simulink model "MAGLEV_StateSpace_szabalyozo"  (Simulink 7.4)
settings: Solver=ode45  StartTime=0.0  StopTime=15  FixedStep=0.01  RelTol=1e-3
undefined symbols (not defined in the file): C, F, G, g, H, K, L0, m, magnitude, Nu, Nx, Q, R, u0, x01, x02, x03
settings Model: Creator=Fodi  LastModifiedBy=Fodi

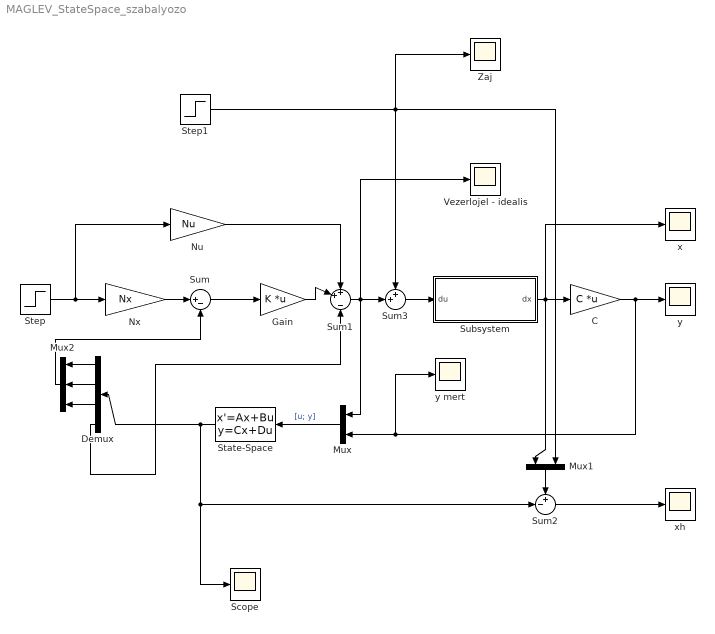
== system MAGLEV_StateSpace_szabalyozo ==
  C : Gain  Gain=C  Multiplication=Matrix(K*u)  ParameterDataType=fixdt(1, 16)  ParameterScaling=2^0  OutDataType=fixdt(1, 16)  OutScaling=2^0
  Demux : Demux
  Gain : Gain  Gain=K  Multiplication=Matrix(K*u)  ParameterDataType=fixdt(1, 16)  ParameterScaling=2^0  OutDataType=fixdt(1, 16)  OutScaling=2^0
  Mux : Mux  Inputs=2
  Mux1 : Mux  Inputs=2
  Mux2 : Mux  Inputs=3
  Nu : Gain  Gain=Nu  ParameterDataType=fixdt(1, 16)  ParameterScaling=2^0  OutDataType=fixdt(1, 16)  OutScaling=2^0
  Nx : Gain  Gain=Nx  ParameterDataType=fixdt(1, 16)  ParameterScaling=2^0  OutDataType=fixdt(1, 16)  OutScaling=2^0
  Scope : Scope
      settings: SaveName=xb
  State-Space : StateSpace  A=F  B=[H G]  C=eye(size(F))  D=zeros(size(F,1),size([H G],2))
  Step : Step  Time=0  After=0.001  SampleTime=0
  Step1 : Step  Time=2  After=0  SampleTime=0
  Subsystem : Subsystem
  Sum : Sum  Inputs=|+-  OutDataType=fixdt(1, 16)  OutScaling=2^0
  Sum1 : Sum  Inputs=++|-  OutDataType=fixdt(1, 16)  OutScaling=2^0
  Sum2 : Sum  Inputs=+-|  OutDataType=fixdt(1, 16)  OutScaling=2^0
  Sum3 : Sum  Inputs=++|  OutDataType=fixdt(1, 16)  OutScaling=2^0
  Vezerlojel - idealis : Scope
      settings: TimeRange=10  YMin=-1  YMax=3  SaveName=u
  Zaj : Scope
      settings: SaveName=ScopeData2
  x : Scope
      settings: SaveName=x
  xh : Scope
      settings: TimeRange=10  YMin=-0.02  YMax=0.12
  y : Scope
      settings: TimeRange=10  YMin=0  YMax=0.0025  SaveName=y
  y mert : Scope
      settings: TimeRange=5  YMin=0  YMax=0.003  SaveName=ym
  wires:
  Step/1 -> Nx/1, Nu/1
  Nx/1 -> Sum/1
  Nu/1 -> Sum1/1
  Gain/1 -> Sum1/2
  Sum/1 -> Gain/1
  Sum1/1 -> Mux/1, Sum3/2, Vezerlojel - idealis/1
  Subsystem/1(dx) -> C/1, Mux1/1, x/1
  State-Space/1 -> Demux/1, Sum2/2, Scope/1
  Mux/1 -> State-Space/1  "[u; y]"
  Step1/1 -> Sum3/1, Mux1/2, Zaj/1
  Sum3/1 -> Subsystem/1(du)
  Mux1/1 -> Sum2/1
  Mux2/1 -> Sum/2
  Demux/4 -> Sum1/3
  Demux/1 -> Mux2/1
  Demux/2 -> Mux2/2
  Demux/3 -> Mux2/3
  Sum2/1 -> xh/1
  C/1 -> y/1, Mux/2, y mert/1

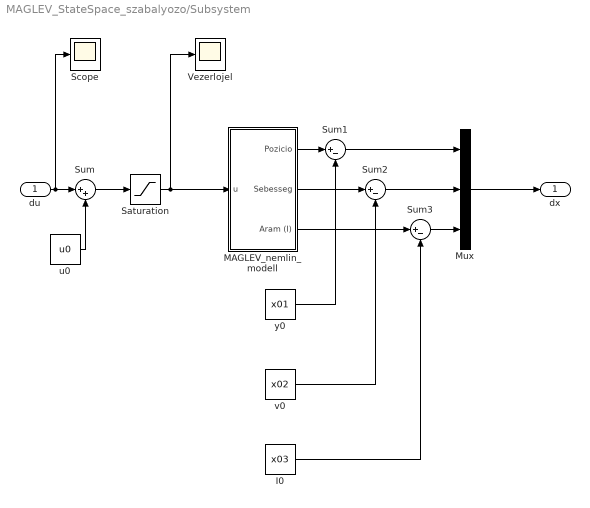
== system MAGLEV_StateSpace_szabalyozo/Subsystem ==
  du : Inport  OutDataType=fixdt(1, 16)  OutScaling=2^0
  I0 : Constant  Value=x03  OutDataType=fixdt(1, 16)  OutScaling=2^0
  MAGLEV_nemlin_modell : Subsystem
  Mux : Mux  Inputs=3
  Saturation : Saturate  UpperLimit=30  LowerLimit=-30  OutDataType=fixdt(1, 16)  OutScaling=2^0
  Scope : Scope
  Sum : Sum  Inputs=|++  OutDataType=fixdt(1, 16)  OutScaling=2^0
  Sum1 : Sum  Inputs=|+-  OutDataType=fixdt(1, 16)  OutScaling=2^0
  Sum2 : Sum  Inputs=|+-  OutDataType=fixdt(1, 16)  OutScaling=2^0
  Sum3 : Sum  Inputs=|+-  OutDataType=fixdt(1, 16)  OutScaling=2^0
  Vezerlojel : Scope
      settings: TimeRange=10  YMin=11  YMax=16  SaveName=ScopeData3
  u0 : Constant  Value=u0  OutDataType=fixdt(1, 16)  OutScaling=2^0
  v0 : Constant  Value=x02  OutDataType=fixdt(1, 16)  OutScaling=2^0
  y0 : Constant  Value=x01  OutDataType=fixdt(1, 16)  OutScaling=2^0
  dx : Outport  OutDataType=fixdt(1, 16)  OutScaling=2^0
  wires:
  y0/1 -> Sum1/2
  v0/1 -> Sum2/2
  I0/1 -> Sum3/2
  MAGLEV_nemlin_modell/3(Aram (I)) -> Sum3/1
  Sum3/1 -> Mux/3
  Sum2/1 -> Mux/2
  Sum1/1 -> Mux/1
  u0/1 -> Sum/2
  Mux/1 -> dx/1
  MAGLEV_nemlin_modell/2(Sebesseg) -> Sum2/1
  MAGLEV_nemlin_modell/1(Pozicio) -> Sum1/1
  du/1 -> Scope/1, Sum/1
  Sum/1 -> Saturation/1
  Saturation/1 -> MAGLEV_nemlin_modell/1(u), Vezerlojel/1

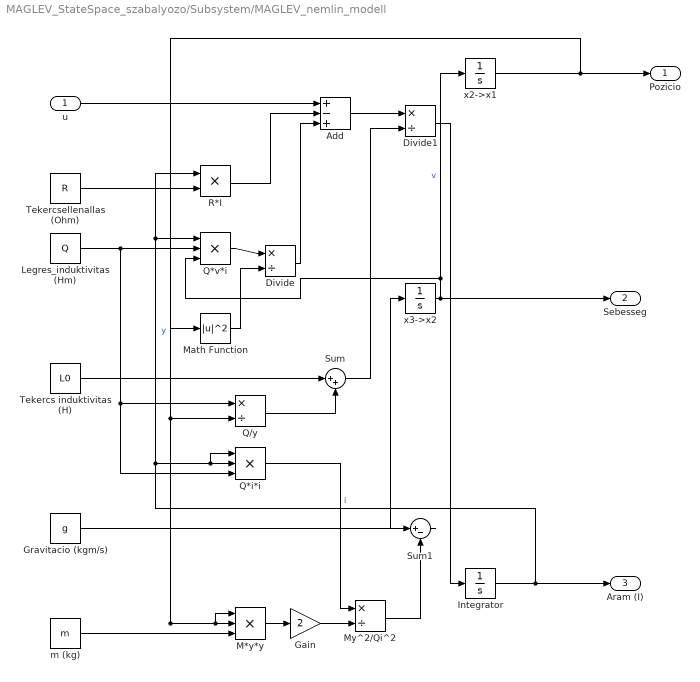
== system MAGLEV_StateSpace_szabalyozo/Subsystem/MAGLEV_nemlin_modell ==
  u : Inport  Tag=v  OutDataType=fixdt(1, 16)  OutScaling=2^0
  Add : Sum  Inputs=+-+  OutDataType=fixdt(1, 16)  OutScaling=2^-10
  Divide : Product  Inputs=*/  OutDataType=fixdt(1, 16)  OutScaling=2^-10
  Divide1 : Product  Inputs=*/  OutDataType=fixdt(1, 16)  OutScaling=2^-10
  Gain : Gain  Gain=2  ParameterDataType=fixdt(1, 16)  ParameterScaling=2^0  OutDataType=fixdt(1, 16)  OutScaling=2^0
  Gravitacio (kgm/s) : Constant  Value=g  OutDataType=fixdt(1, 16)  OutScaling=2^0
  Integrator : Integrator  InitialCondition=x03
  Legres_induktivitas (Hm) : Constant  Value=Q  OutDataType=fixdt(1, 16)  OutScaling=2^0
  M*y*y : Product  Inputs=3  OutDataType=fixdt(1, 16)  OutScaling=2^0  RndMeth=Zero
  Math Function : Math  Operator=magnitude^2  OutDataType=fixdt(1, 16)  OutScaling=2^0  SaturateOnIntegerOverflow=on
  My^2/Qi^2 : Product  Inputs=*/  OutDataType=fixdt(1, 16)  OutScaling=2^-10
  Q*i*i : Product  Inputs=3  OutDataType=fixdt(1, 16)  OutScaling=2^0  RndMeth=Zero
  Q*v*i : Product  Inputs=3  OutDataType=fixdt(1, 16)  OutScaling=2^0  RndMeth=Zero
  Q/y : Product  Inputs=*/  OutDataType=fixdt(1, 16)  OutScaling=2^-10
  R*I : Product  OutDataType=fixdt(1, 16)  OutScaling=2^0  RndMeth=Zero
  Sum : Sum  Inputs=|++  OutDataType=fixdt(1, 16)  OutScaling=2^0
  Sum1 : Sum  Inputs=|+-  OutDataType=fixdt(1, 16)  OutScaling=2^0
  Tekercs induktivitas (H) : Constant  Value=L0  OutDataType=fixdt(1, 16)  OutScaling=2^0
  Tekercsellenallas (Ohm) : Constant  Value=R  OutDataType=fixdt(1, 16)  OutScaling=2^0
  m (kg) : Constant  Value=m  OutDataType=fixdt(1, 16)  OutScaling=2^0
  x2->x1 : Integrator  InitialCondition=x01
  x3->x2 : Integrator  InitialCondition=0.01
  Pozicio : Outport  OutDataType=fixdt(1, 16)  OutScaling=2^0
  Sebesseg : Outport  Port=2  OutDataType=fixdt(1, 16)  OutScaling=2^0
  Aram (I) : Outport  Port=3  OutDataType=fixdt(1, 16)  OutScaling=2^0
  wires:
  x2->x1/1 -> Pozicio/1, Q/y/2, Math Function/1, M*y*y/2, M*y*y/1  "y"
  Sum1/1 -> x3->x2/1
  Gravitacio (kgm/s)/1 -> Sum1/1
  My^2/Qi^2/1 -> Sum1/2
  Gain/1 -> My^2/Qi^2/2
  M*y*y/1 -> Gain/1
  Sum/1 -> Divide1/2
  Tekercs induktivitas (H)/1 -> Sum/1
  Q/y/1 -> Sum/2
  Math Function/1 -> Divide/2
  Divide/1 -> Add/3
  Q*v*i/1 -> Divide/1
  R*I/1 -> Add/2
  Divide1/1 -> Integrator/1
  Add/1 -> Divide1/1
  u/1 -> Add/1
  m (kg)/1 -> M*y*y/3
  Legres_induktivitas (Hm)/1 -> Q*v*i/2, Q/y/1, Q*i*i/3
  Tekercsellenallas (Ohm)/1 -> R*I/2
  Q*i*i/1 -> My^2/Qi^2/1
  x3->x2/1 -> Q*v*i/3, x2->x1/1, Sebesseg/1  "v"
  Integrator/1 -> Aram (I)/1, Q*i*i/2, Q*i*i/1, Q*v*i/1, R*I/1  "i"
